simulink model "Fuzzy_PID"  (R2018a)
settings: Solver=VariableStepAuto  StartTime=0.0  StopTime=1000  RelTol=1e-3
libraries: simulink x2, fuzblock x1
settings Model: Creator=lazyn  LastModifiedBy=lazyn
settings SolverCC: AlgebraicLoopSolver=LineSearch

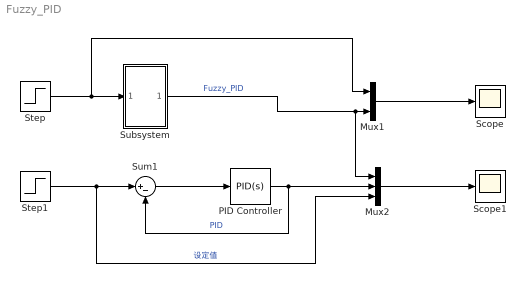
== system Fuzzy_PID ==
  Mux1 : Mux  Inputs=2
  Mux2 : Mux  Inputs=3
  PID Controller : simulink/Continuous/PID Controller  Controller=PID  TimeDomain=Continuous-time  SampleTime=-1  IntegratorMethod=Forward Euler  FilterMethod=Forward Euler  Form=Parallel  UseFilter=on  ControllerParametersSource=internal  P=0.05  I=0.01  D=0.005  N=100  InitialConditionSource=internal  InitialConditionForIntegrator=0  InitialConditionForFilter=0  ExternalReset=none  LimitOutput=off  UpperSaturationLimit=inf  LowerSaturationLimit=-inf  LinearizeAsGain=on  AntiWindupMode=none  Kb=1  TrackingMode=off  Kt=1  PParamMin=[]  PParamMax=[]  IParamMin=[]  IParamMax=[]  DParamMin=[]  DParamMax=[]  NParamMin=[]  NParamMax=[]  KbParamMin=[]  KbParamMax=[]  KtParamMin=[]  KtParamMax=[]  POutMin=[]  POutMax=[]  IOutMin=[]  IOutMax=[]  DOutMin=[]  DOutMax=[]  NOutMin=[]  NOutMax=[]  KbOutMin=[]  KbOutMax=[]  KtOutMin=[]  KtOutMax=[]  IntegratorOutMin=[]  IntegratorOutMax=[]  FilterOutMin=[]  FilterOutMax=[]  SumOutMin=[]  SumOutMax=[]  SumI1OutMin=[]  SumI1OutMax=[]  SumI2OutMin=[]  SumI2OutMax=[]  SumI3OutMin=[]  SumI3OutMax=[]  SumDOutMin=[]  SumDOutMax=[]  SaturationOutMin=[]  SaturationOutMax=[]  IntegratorContinuousStateAttributes=''  IntegratorStateMustResolveToSignalObject=off  IntegratorRTWStateStorageClass=Auto  FilterContinuousStateAttributes=''  FilterStateMustResolveToSignalObject=off  FilterRTWStateStorageClass=Auto  DifferentiatorICPrevScaledInput=0  DifferentiatorOutMin=[]  DifferentiatorOutMax=[]  FilterDiffOutCoefMin=[]  FilterDiffOutCoefMax=[]  SumDenOutMin=[]  SumDenOutMax=[]  SumNumOutMin=[]  SumNumOutMax=[]  ReciprocalOutMin=[]  ReciprocalOutMax=[]  DivideOutMin=[]  DivideOutMax=[]  TunerSelectOption=Transfer Function Based (PID Tuner App)
  Scope : Scope
  Scope1 : Scope
  Step : Step  Time=0  After=110  SampleTime=0
  Step1 : Step  Time=0  After=110  SampleTime=0
  Subsystem : Subsystem
  Sum1 : Sum  Inputs=|+-
  wires:
  Step1/1 -> Mux2/3, Sum1/1  "设定值"
  Subsystem/1(Out1) -> Mux2/1, Mux1/2  "Fuzzy_PID"
  Mux1/1 -> Scope/1
  PID Controller/1 -> Sum1/2, Mux2/2  "PID"
  Mux2/1 -> Scope1/1
  Sum1/1 -> PID Controller/1
  Step/1 -> Mux1/1, Subsystem/1(In1)

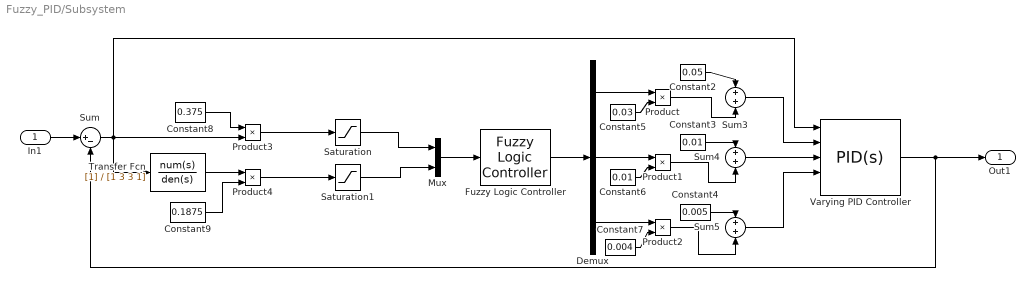
== system Fuzzy_PID/Subsystem ==
  In1 : Inport
  Constant2 : Constant  Value=0.05
  Constant3 : Constant  Value=0.01
  Constant4 : Constant  Value=0.005
  Constant5 : Constant  Value=0.03
  Constant6 : Constant  Value=0.01
  Constant7 : Constant  Value=0.004
  Constant8 : Constant  Value=0.375
  Constant9 : Constant  Value=0.1875
  Demux : Demux  Outputs=3
  Fuzzy Logic Controller : fuzblock/Fuzzy Logic  Controller  FIS=Fuzzy_PID  OutputSampleNumber=101  DataType=double  FuzzifiedInputs=off  RuleFiringStrengths=off  RuleOutputs=off  AggregatedOutputs=off  SimulateUsing=Interpreted execution  OutOfRangeInputValueMessage=warning  NoRuleFiredMessage=warning  EmptyOutputFuzzySetMessage=warning
  Mux : Mux  Inputs=2
  Product{,1..4} (5 alike) : Product
  Saturation : Saturate  UpperLimit=3  LowerLimit=-3
  Saturation1 : Saturate  UpperLimit=3  LowerLimit=-3
  Sum : Sum  Inputs=|+-
  Sum3 : Sum
  Sum4 : Sum
  Sum5 : Sum
  Transfer Fcn : TransferFcn  Denominator=[1 3 3 1]
  Varying PID Controller : simulink/Continuous/PID Controller  Controller=PID  TimeDomain=Continuous-time  SampleTime=-1  IntegratorMethod=Forward Euler  FilterMethod=Forward Euler  Form=Parallel  UseFilter=on  ControllerParametersSource=external  P=1  I=1  D=0  N=100  InitialConditionSource=internal  InitialConditionForIntegrator=0  InitialConditionForFilter=0  ExternalReset=none  LimitOutput=off  UpperSaturationLimit=inf  LowerSaturationLimit=-inf  LinearizeAsGain=on  AntiWindupMode=none  Kb=1  TrackingMode=off  Kt=1  PParamMin=[]  PParamMax=[]  IParamMin=[]  IParamMax=[]  DParamMin=[]  DParamMax=[]  NParamMin=[]  NParamMax=[]  KbParamMin=[]  KbParamMax=[]  KtParamMin=[]  KtParamMax=[]  POutMin=[]  POutMax=[]  IOutMin=[]  IOutMax=[]  DOutMin=[]  DOutMax=[]  NOutMin=[]  NOutMax=[]  KbOutMin=[]  KbOutMax=[]  KtOutMin=[]  KtOutMax=[]  IntegratorOutMin=[]  IntegratorOutMax=[]  FilterOutMin=[]  FilterOutMax=[]  SumOutMin=[]  SumOutMax=[]  SumI1OutMin=[]  SumI1OutMax=[]  SumI2OutMin=[]  SumI2OutMax=[]  SumI3OutMin=[]  SumI3OutMax=[]  SumDOutMin=[]  SumDOutMax=[]  SaturationOutMin=[]  SaturationOutMax=[]  IntegratorContinuousStateAttributes=''  IntegratorStateMustResolveToSignalObject=off  IntegratorRTWStateStorageClass=Auto  FilterContinuousStateAttributes=''  FilterStateMustResolveToSignalObject=off  FilterRTWStateStorageClass=Auto  DifferentiatorICPrevScaledInput=0  DifferentiatorOutMin=[]  DifferentiatorOutMax=[]  InitialConditionSetting=State (most efficient)  FilterDiffOutCoefMin=[]  FilterDiffOutCoefMax=[]  SumDenOutMin=[]  SumDenOutMax=[]  SumNumOutMin=[]  SumNumOutMax=[]  ReciprocalOutMin=[]  ReciprocalOutMax=[]  DivideOutMin=[]  DivideOutMax=[]  TunerSelectOption=Transfer Function Based (PID Tuner App)
  Out1 : Outport
  wires:
  Demux/2 -> Product1/1
  Saturation1/1 -> Mux/2
  Transfer Fcn/1 -> Product4/1
  Sum/1 -> Transfer Fcn/1, Product3/2, Varying PID Controller/1
  Constant4/1 -> Sum5/1
  In1/1 -> Sum/1
  Constant5/1 -> Product/2
  Constant2/1 -> Sum3/1
  Constant9/1 -> Product4/2
  Constant3/1 -> Sum4/1
  Product3/1 -> Saturation/1
  Product1/1 -> Sum4/2
  Varying PID Controller/1 -> Out1/1, Sum/2
  Product/1 -> Sum3/2
  Constant6/1 -> Product1/2
  Sum3/1 -> Varying PID Controller/2
  Mux/1 -> Fuzzy Logic Controller/1
  Fuzzy Logic Controller/1 -> Demux/1
  Constant7/1 -> Product2/2
  Demux/1 -> Product/1
  Sum5/1 -> Varying PID Controller/4
  Demux/3 -> Product2/1
  Sum4/1 -> Varying PID Controller/3
  Saturation/1 -> Mux/1
  Constant8/1 -> Product3/1
  Product2/1 -> Sum5/2
  Product4/1 -> Saturation1/1
